simulink model "positionWalking_legacy"  (Simulink 8.3)
settings: Solver=FixedStepDiscrete  StartTime=0.0  StopTime=Config.t_end  FixedStep=Config.t_step  RelTol=1e-3
InitFcn:
  | cd(fileparts(which(bdroot)));
  | initTorqueWalking;
undefined symbols (not defined in the file): Config, DiscIntNeverNeededParam, gains, ROBOT_DOF
libraries: WBToolboxLibrary x88
(part 3 of 3)

== matlab function Dynamics and Kinematics/Inverse Kinematics/Compute tasks accelerations ==
  data: pos_vel_acc_CoM_des input double; acc_task_star output double; pose_vel_acc_LFoot_des input double; pose_vel_acc_RFoot_des input double; orient_vel_acc_Rot_task_des input double; pos_vel_CoM input double; pose_vel_LFoot input double; pose_vel_RFoot input double; orient_vel_Rot_task input double; Kp_Kd_CoM input double; Kp_Kd_LFoot input double; Kp_Kd_RFoot input double; Kp_Kd_Rot_task input double; feetInContact input double; Sat parameter double
function acc_task_star = setTasksAccelerationsFCN(pos_vel_acc_CoM_des,pose_vel_acc_LFoot_des,pose_vel_acc_RFoot_des,orient_vel_acc_Rot_task_des, ...
                                                  pos_vel_CoM, pose_vel_LFoot, pose_vel_RFoot, orient_vel_Rot_task, ...
                                                  Kp_Kd_CoM, Kp_Kd_LFoot, Kp_Kd_RFoot, Kp_Kd_Rot_task, feetInContact, Sat) 

    acc_task_star = setTasksAccelerations(pos_vel_acc_CoM_des,pose_vel_acc_LFoot_des,pose_vel_acc_RFoot_des,orient_vel_acc_Rot_task_des, ...
                                          pos_vel_CoM, pose_vel_LFoot, pose_vel_RFoot, orient_vel_Rot_task, ...
                                          Kp_Kd_CoM, Kp_Kd_LFoot, Kp_Kd_RFoot, Kp_Kd_Rot_task, feetInContact, Sat);   
end

== matlab function Dynamics and Kinematics/Inverse Kinematics/ComputeTasksPoseAndVelocity/Compose Task Pose and Velocity ==
  data: vel_CoM input double; vel_LFoot input double; vel_RFoot input double; vel_Rot_task input double; pos_vel_CoM output double; pose_vel_LFoot output double; pose_vel_RFoot output double; orient_vel_Rot_task output double; w_H_CoM input double; w_H_l_sole input double; w_H_r_sole input double; w_H_Rot_task input double
function [pos_vel_CoM, pose_vel_LFoot, pose_vel_RFoot, orient_vel_Rot_task] = ...
             composeTaskPoseAndVelocityFCN(vel_CoM, vel_LFoot, vel_RFoot, vel_Rot_task, ...
                                           w_H_CoM, w_H_l_sole, w_H_r_sole, w_H_Rot_task)
                                                                                                                              
    [pos_vel_CoM, pose_vel_LFoot, pose_vel_RFoot, orient_vel_Rot_task] = ...
       composeTaskPoseAndVelocity(vel_CoM, vel_LFoot, vel_RFoot, vel_Rot_task, ...
                                  w_H_CoM, w_H_l_sole, w_H_r_sole, w_H_Rot_task);
end

== matlab function Dynamics and Kinematics/Task Accelerations/Compute tasks accelerations ==
  data: pos_vel_acc_CoM_des input double; acc_task_star output double; pose_vel_acc_LFoot_des input double; pose_vel_acc_RFoot_des input double; orient_vel_acc_Rot_task_des input double; pos_vel_CoM input double; pose_vel_LFoot input double; pose_vel_RFoot input double; orient_vel_Rot_task input double; Kp_Kd_CoM input double; Kp_Kd_LFoot input double; Kp_Kd_RFoot input double; Kp_Kd_Rot_task input double; feetInContact input double; Sat parameter double
function acc_task_star = setTasksAccelerationsFCN(pos_vel_acc_CoM_des,pose_vel_acc_LFoot_des,pose_vel_acc_RFoot_des,orient_vel_acc_Rot_task_des, ...
                                                  pos_vel_CoM, pose_vel_LFoot, pose_vel_RFoot, orient_vel_Rot_task, ...
                                                  Kp_Kd_CoM, Kp_Kd_LFoot, Kp_Kd_RFoot, Kp_Kd_Rot_task, feetInContact, Sat) 

    acc_task_star = setTasksAccelerations(pos_vel_acc_CoM_des,pose_vel_acc_LFoot_des,pose_vel_acc_RFoot_des,orient_vel_acc_Rot_task_des, ...
                                          pos_vel_CoM, pose_vel_LFoot, pose_vel_RFoot, orient_vel_Rot_task, ...
                                          Kp_Kd_CoM, Kp_Kd_LFoot, Kp_Kd_RFoot, Kp_Kd_Rot_task, feetInContact, Sat); 
end

== matlab function Dynamics and Kinematics/Task Accelerations/ComputeTasksPoseAndVelocity/Compose Task Pose and Velocity ==
  data: vel_CoM input double; vel_LFoot input double; vel_RFoot input double; vel_Rot_task input double; pos_vel_CoM output double; pose_vel_LFoot output double; pose_vel_RFoot output double; orient_vel_Rot_task output double; w_H_CoM input double; w_H_l_sole input double; w_H_r_sole input double; w_H_Rot_task input double
function [pos_vel_CoM, pose_vel_LFoot, pose_vel_RFoot, orient_vel_Rot_task] = ...
             composeTaskPoseAndVelocityFCN(vel_CoM, vel_LFoot, vel_RFoot, vel_Rot_task, ...
                                           w_H_CoM, w_H_l_sole, w_H_r_sole, w_H_Rot_task)
                                                                                                                              
    [pos_vel_CoM, pose_vel_LFoot, pose_vel_RFoot, orient_vel_Rot_task] = ...
        composeTaskPoseAndVelocity(vel_CoM, vel_LFoot, vel_RFoot, vel_Rot_task, ...
                                   w_H_CoM, w_H_l_sole, w_H_r_sole, w_H_Rot_task);
end

== matlab function Robot State and References/Gain Scheduling/Gain scheduling Function ==
  data: state input double; Kp_CoM output double; Kd_CoM output double; Kp_LFoot output double; Kd_LFoot output double; Kp_RFoot output double; Kd_RFoot output double; Kp_Rot_task output double; Kd_Rot_task output double; impedances output double; dampings output double; gains parameter double
function [Kp_CoM, Kd_CoM, Kp_LFoot, Kd_LFoot, Kp_RFoot, Kd_RFoot, Kp_Rot_task, Kd_Rot_task, impedances, dampings] = gainSchedulingFCN(state,gains)

    [Kp_CoM, Kd_CoM, Kp_LFoot, Kd_LFoot, Kp_RFoot, Kd_RFoot, Kp_Rot_task, Kd_Rot_task, impedances, dampings] = gainScheduling(state,gains);
end

== matlab function Robot State and References/Reference Velocities and Accelerations/Reference Orientations/Compute Reference Angular Accelerations ==
  data: w_R_LFoot_des input double; w_R_RFoot_des input double; w_R_Rot_task_des input double; w_R_LFoot input double; w_R_RFoot input double; omegaDot_LFoot output double; omegaDot_RFoot output double; omegaDot_Rot_task output double; w_R_Rot_task input double; omega_LFoot input double; omega_RFoot input double; omega_Rot_task input double; Config parameter double
function [omegaDot_LFoot, omegaDot_RFoot, omegaDot_Rot_task] = computeRefAngAccelerationFCN(w_R_LFoot_des, w_R_RFoot_des, w_R_Rot_task_des, w_R_LFoot, w_R_RFoot, w_R_Rot_task, ...
                                                                                            omega_LFoot, omega_RFoot, omega_Rot_task, Config)
         
    % Compute reference angular accelerations given a desired rotation matrix
    omegaDot_LFoot     = rotationalPID(w_R_LFoot, omega_LFoot, w_R_LFoot_des, zeros(3,1), zeros(3,1), Config.t_smoothingTimeRotation, Config.t_smoothingTimeAngVel);
    omegaDot_RFoot     = rotationalPID(w_R_RFoot, omega_RFoot, w_R_RFoot_des, zeros(3,1), zeros(3,1), Config.t_smoothingTimeRotation, Config.t_smoothingTimeAngVel);
    omegaDot_Rot_task  = rotationalPID(w_R_Rot_task, omega_Rot_task, w_R_Rot_task_des, zeros(3,1), zeros(3,1), Config.t_smoothingTimeRotation, Config.t_smoothingTimeAngVel);
end

== matlab function Robot State and References/State Machine/Select Current State and References/State Machines ==
  data: s_0 input double; w_H_CoM_0 input double; w_H_LFoot_0 input double; w_H_RFoot_0 input double; w_H_Rot_task_0 input double; w_H_fixed_LFoot input double; w_H_fixed_RFoot input double; t input double; state output double; references_CoM output double; references_LFoot output double; references_RFoot output double; references_RotTask output double; feetInContact output double; references_s output double; w_H_b output double; Config parameter double
function [state, references_CoM, references_LFoot, references_RFoot, references_RotTask, feetInContact, references_s, w_H_b] = stateMachineFCN ...
                 (s_0, w_H_CoM_0, w_H_LFoot_0, w_H_RFoot_0, w_H_Rot_task_0, w_H_fixed_LFoot, w_H_fixed_RFoot, t, Config)

    % Collection of state machines. Currently available: 
    %
    %    internalCoordinator 
    %
    [state, references_CoM, references_LFoot, references_RFoot, references_RotTask, feetInContact, references_s, w_H_b] = internalCoordinator ...
             (s_0, w_H_CoM_0, w_H_LFoot_0, w_H_RFoot_0, w_H_Rot_task_0, w_H_fixed_LFoot, w_H_fixed_RFoot, t, Config);
end

== matlab function Robot State and References/State Machine/World to fixed link transform/w_H_b with left foot fixed/fromImuToHomogeousTransformFCN ==
  data: imu_H_link input double; imu_H_link_0 input double; link_H_base input double; inertial_0 input double; inertial input double; neck_pos input double; w_H_b output double; Config parameter double
function w_H_b = worldToBaseTransformWithIMUFCN(imu_H_link,imu_H_link_0,link_H_base,inertial_0,inertial,neck_pos,Config)

    w_H_b = worldToBaseTransformWithIMU(imu_H_link,imu_H_link_0,link_H_base,inertial_0,inertial,neck_pos,Config);

end

== matlab function Robot State and References/State Machine/World to fixed link transform/w_H_b with right foot fixed/fromImuToHomogeousTransformFCN ==
  data: imu_H_link input double; imu_H_link_0 input double; link_H_base input double; inertial_0 input double; inertial input double; neck_pos input double; w_H_b output double; Config parameter double
function w_H_b = worldToBaseTransformWithIMUFCN(imu_H_link,imu_H_link_0,link_H_base,inertial_0,inertial,neck_pos,Config)

    w_H_b = worldToBaseTransformWithIMU(imu_H_link,imu_H_link_0,link_H_base,inertial_0,inertial,neck_pos,Config);

end

== matlab function Robot State and References/Reference Velocities and Accelerations/Reference Orientations/Compute Rotation Matrix Derivative ==
  data: RDot_LFoot output double; RDot_RFoot output double; RDot_Rot_task output double; omega_LFoot input double; omega_RFoot input double; omega_Rot_task input double; w_R_LFoot input double; w_R_RFoot input double; w_R_Rot_task input double
function [RDot_LFoot, RDot_RFoot, RDot_Rot_task] = rotationDerivativeFromAngVelFCN(omega_LFoot, omega_RFoot, omega_Rot_task, w_R_LFoot, w_R_RFoot, w_R_Rot_task)
         
    % Compute the rotation matrix derivative given the angular velocity
    RDot_LFoot     = rotationDerivativeFromAngVel(omega_LFoot,w_R_LFoot);
    RDot_RFoot     = rotationDerivativeFromAngVel(omega_RFoot,w_R_RFoot);
    RDot_Rot_task  = rotationDerivativeFromAngVel(omega_Rot_task, w_R_Rot_task);
       
end

== matlab function Robot State and References/State Machine/compute state velocity/Compute Base Velocity ==
  data: J_LeftFoot input double; J_RightFoot input double; feetInContact input double; nu_b output double; sDot input double; Sat parameter double
function nu_b = computeBaseVelocityFCN(J_LeftFoot,J_RightFoot, feetInContact, sDot, Sat)

    nu_b = computeBaseVelocity(J_LeftFoot,J_RightFoot, feetInContact, sDot, Sat);
end

== matlab function Dynamics and Kinematics/Inverse Kinematics/QP-Based Inverse Kinematics/inverse kinematics integration/Rewrite Base Pose as transformation matrix ==
  data: q_quat input double; q_transf output double
function q_transf = fromQuaternionsToTransfMatrFCN(q_quat)

    % converts the floating base pose from a quaternion representation 
    % [7 + ROBOT_DOF * 1]to a tranformation matrix rapresentation 
    % [16 + ROBOT_DOF * 1]
    q_transf = fromQuaternionsToTransfMatr(q_quat);

end

== matlab function Dynamics and Kinematics/Inverse Kinematics/QP-Based Inverse Kinematics/inverse kinematics integration/Compute Base Pose Derivative ==
  data: nu_b input double; pose_bDot output double; pose_b input double
function pose_bDot = basePoseDerivativeFCN(nu_b, pose_b)

    % time derivative of the floating base pose
    pose_bDot = basePoseDerivative(nu_b, pose_b);
end

== matlab function Dynamics and Kinematics/Inverse Kinematics/QP-Based Inverse Kinematics/inverse kinematics integration/Rewrite Base Pose as pos+quat ==
  data: q_transf input double; q_quat output double
function q_quat = fromTransfMatrixToQuaternionsFCN(q_transf)

    % converts the state position expresed in terms of transformation matrix 
    % [16 + ROBOT_DOF * 1] to quaternion representation [7 + ROBOT_DOF * 1] 
    q_quat = fromTransfMatrixToQuaternions(q_transf);

end
